simulink model "Attitude"  (R2023b)
settings: Solver=VariableStepAuto  StartTime=0.0  StopTime=10.0  RelTol=1e-3
values from neighbouring files (symbols this model uses):
  gravity = Airplane_data(52)    [Data_edit.m]
libraries: simulink_extras x6, slpidlib x3
settings Model: Creator=saifg  LastModifiedBy=saifg

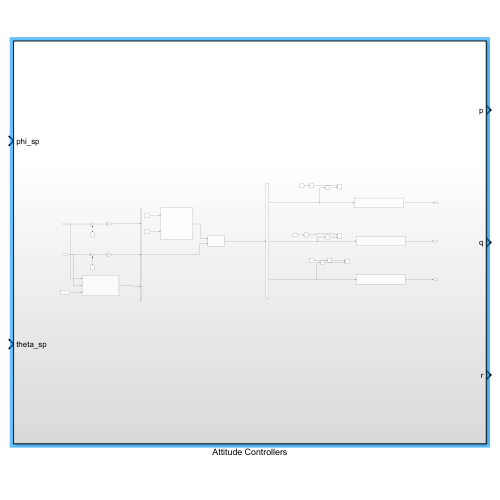
[thumbnail: Simulink's stored preview of the top-level diagram]
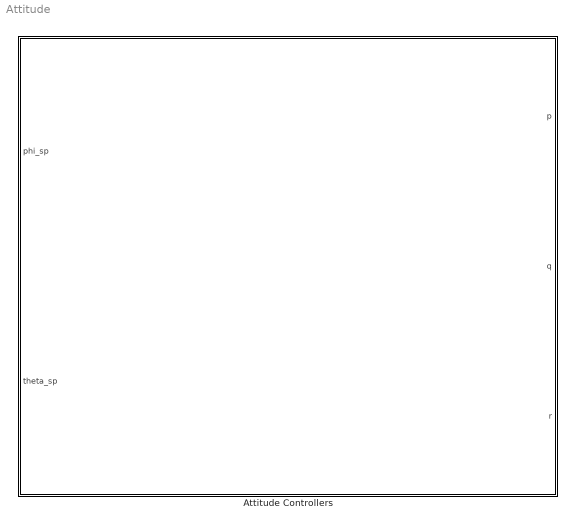
== system Attitude ==
  Attitude Controllers : Subsystem

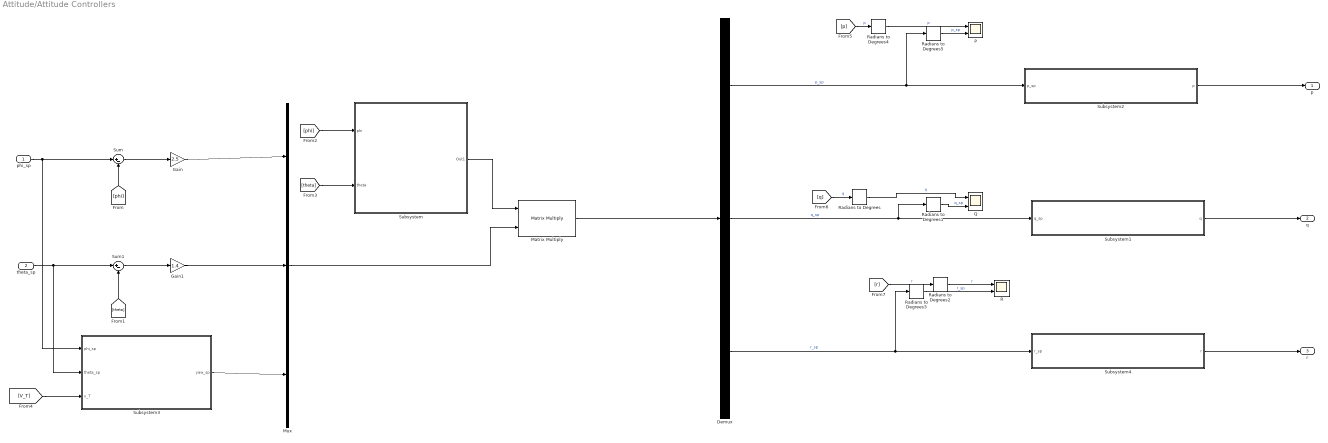
== system Attitude/Attitude Controllers ==
  phi_sp : Inport
  theta_sp : Inport  Port=2
  Demux : Demux  Outputs=3
  Gain : Gain  Gain=2.5
  Gain1 : Gain  Gain=1.4
  Matrix Multiply : Product  Multiplication=Matrix(*)
  Mux : Mux  Inputs=3
  P : Scope  NumInputPorts=2
  Q : Scope  NumInputPorts=2
  R : Scope  NumInputPorts=2
  Radians to Degrees{,1..5} (6 alike) : simulink_extras/Transformations/Radians to Degrees
  Subsystem : Subsystem
  Subsystem1 : Subsystem
  Subsystem2 : Subsystem
  Subsystem3 : Subsystem
  Subsystem4 : Subsystem
  Sum : Sum  Inputs=|+-
  Sum1 : Sum  Inputs=|+-
  p : Outport
  q : Outport  Port=2
  r : Outport  Port=3
  wires:
  [phi] -> Sum/2
  phi_sp/1 -> Subsystem3/1(phi_sp), Sum/1
  Sum/1 -> Gain/1
  theta_sp/1 -> Subsystem3/2(theta_sp), Sum1/1
  [theta] -> Sum1/2
  Sum1/1 -> Gain1/1
  Gain/1 -> Mux/1
  Gain1/1 -> Mux/2
  Subsystem/1(Out1) -> Matrix Multiply/1
  Mux/1 -> Matrix Multiply/2
  Demux/2 -> Radians to Degrees1/1, Subsystem1/1(q_sp)  "q_sp"
  Demux/1 -> Radians to Degrees5/1, Subsystem2/1(p_sp)  "p_sp"
  [phi] -> Subsystem/1(phi)
  [theta] -> Subsystem/2(theta)
  [V_T] -> Subsystem3/3(v_T)
  Subsystem3/1(yaw_sp) -> Mux/3
  Demux/3 -> Radians to Degrees3/1, Subsystem4/1(r_sp)  "r_sp"
  Subsystem2/1(p) -> p/1
  Subsystem1/1(q) -> q/1
  Subsystem4/1(r) -> r/1
  [p] -> Radians to Degrees4/1  "p"
  [q] -> Radians to Degrees/1  "q"
  [r] -> Radians to Degrees2/1  "r"
  Radians to Degrees/1 -> Q/1  "q"
  Radians to Degrees1/1 -> Q/2  "q_sp"
  Radians to Degrees2/1 -> R/1  "r"
  Radians to Degrees3/1 -> R/2  "r_sp"
  Radians to Degrees4/1 -> P/1  "p"
  Radians to Degrees5/1 -> P/2  "p_sp"
  Matrix Multiply/1 -> Demux/1

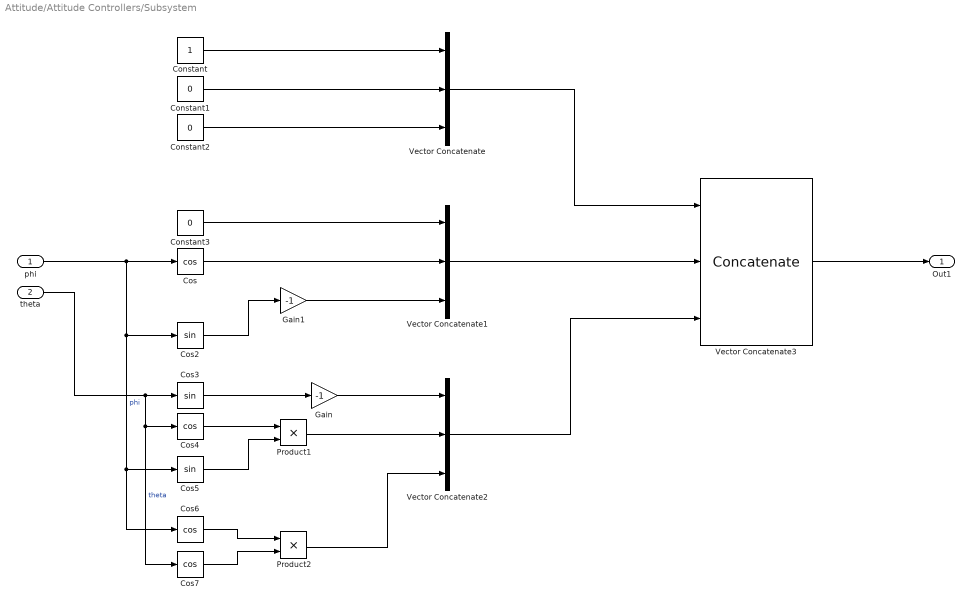
== system Attitude/Attitude Controllers/Subsystem ==
  phi : Inport
  theta : Inport  Port=2
  Constant : Constant
  Constant1 : Constant  Value=0
  Constant2 : Constant  Value=0
  Constant3 : Constant  Value=0
  Cos{,4,6..7} (4 alike) : Trigonometry  Operator=cos
  Cos2 : Trigonometry
  Cos3 : Trigonometry
  Cos5 : Trigonometry
  Gain : Gain  Gain=-1
  Gain1 : Gain  Gain=-1
  Product1 : Product
  Product2 : Product
  Vector Concatenate : Concatenate  NumInputs=3
  Vector Concatenate1 : Concatenate  NumInputs=3
  Vector Concatenate2 : Concatenate  NumInputs=3
  Vector Concatenate3 : Concatenate  NumInputs=3  Mode=Multidimensional array  ConcatenateDimension=2
  Out1 : Outport
  wires:
  Constant2/1 -> Vector Concatenate/3
  Constant1/1 -> Vector Concatenate/2
  Constant/1 -> Vector Concatenate/1
  Constant3/1 -> Vector Concatenate1/1
  Cos/1 -> Vector Concatenate1/2
  Cos2/1 -> Gain1/1
  phi/1 -> Cos6/1, Cos5/1, Cos2/1, Cos/1  "phi"
  theta/1 -> Cos7/1, Cos4/1, Cos3/1  "theta"
  Cos3/1 -> Gain/1
  Gain/1 -> Vector Concatenate2/1
  Cos5/1 -> Product1/2
  Product1/1 -> Vector Concatenate2/2
  Cos4/1 -> Product1/1
  Product2/1 -> Vector Concatenate2/3
  Cos6/1 -> Product2/1
  Cos7/1 -> Product2/2
  Vector Concatenate2/1 -> Vector Concatenate3/3
  Vector Concatenate1/1 -> Vector Concatenate3/2
  Vector Concatenate3/1 -> Out1/1
  Vector Concatenate/1 -> Vector Concatenate3/1
  Gain1/1 -> Vector Concatenate1/3

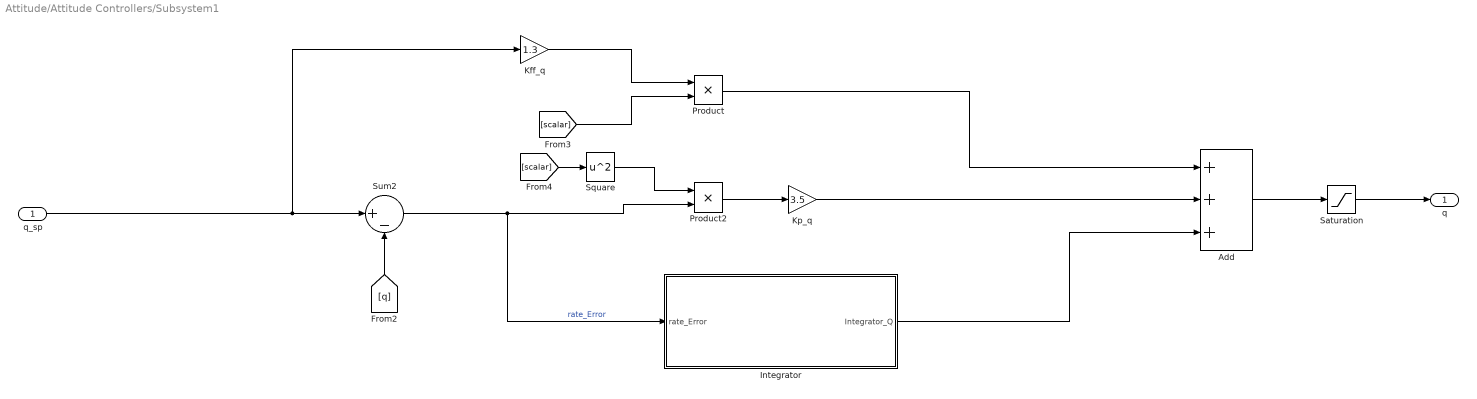
== system Attitude/Attitude Controllers/Subsystem1 ==
  q_sp : Inport
  Add : Sum  Inputs=+++
  Integrator : Subsystem
  Kff_q : Gain  Gain=1.3
  Kp_q : Gain  Gain=3.5
  Product : Product
  Product2 : Product
  Saturation : Saturate  UpperLimit=1  LowerLimit=-1
  Square : Math  Operator=square
  Sum2 : Sum  Inputs=|+-
  q : Outport
  wires:
  Kp_q/1 -> Add/2
  [scalar] -> Product/2
  Square/1 -> Product2/1
  [q] -> Sum2/2
  Kff_q/1 -> Product/1
  q_sp/1 -> Kff_q/1, Sum2/1
  Sum2/1 -> Product2/2, Integrator/1(rate_Error)  "rate_Error"
  [scalar] -> Square/1
  Product2/1 -> Kp_q/1
  Product/1 -> Add/1
  Integrator/1(Integrator_Q) -> Add/3
  Add/1 -> Saturation/1
  Saturation/1 -> q/1

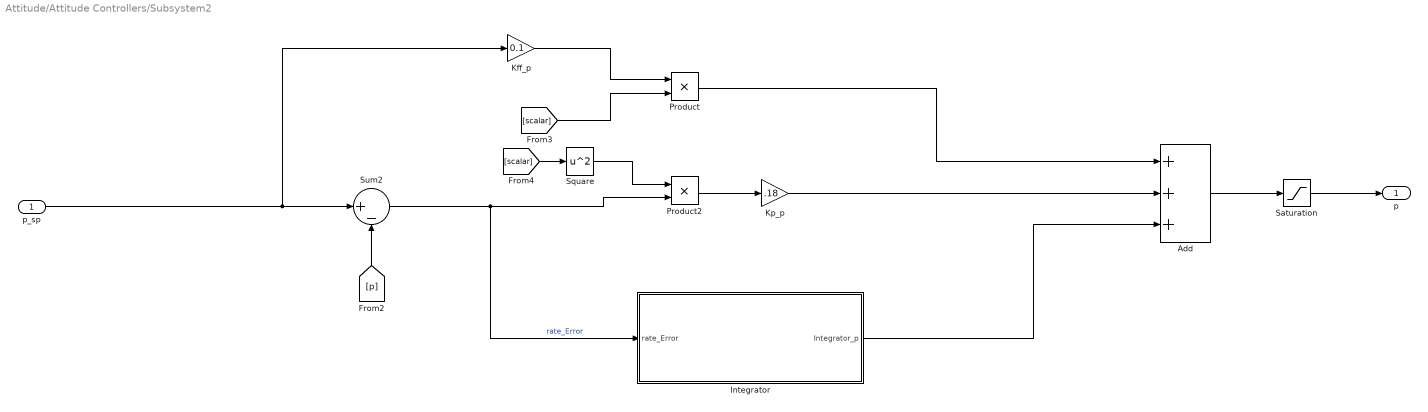
== system Attitude/Attitude Controllers/Subsystem2 ==
  p_sp : Inport
  Add : Sum  Inputs=+++
  Integrator : Subsystem
  Kff_p : Gain  Gain=0.1
  Kp_p : Gain  Gain=.18
  Product : Product
  Product2 : Product
  Saturation : Saturate  UpperLimit=1  LowerLimit=-1
  Square : Math  Operator=square
  Sum2 : Sum  Inputs=|+-
  p : Outport
  wires:
  Add/1 -> Saturation/1
  Integrator/1(Integrator_p) -> Add/3
  Product/1 -> Add/1
  Product2/1 -> Kp_p/1
  [scalar] -> Square/1
  Sum2/1 -> Integrator/1(rate_Error), Product2/2  "rate_Error"
  p_sp/1 -> Sum2/1, Kff_p/1
  Kff_p/1 -> Product/1
  [p] -> Sum2/2
  Square/1 -> Product2/1
  [scalar] -> Product/2
  Kp_p/1 -> Add/2
  Saturation/1 -> p/1

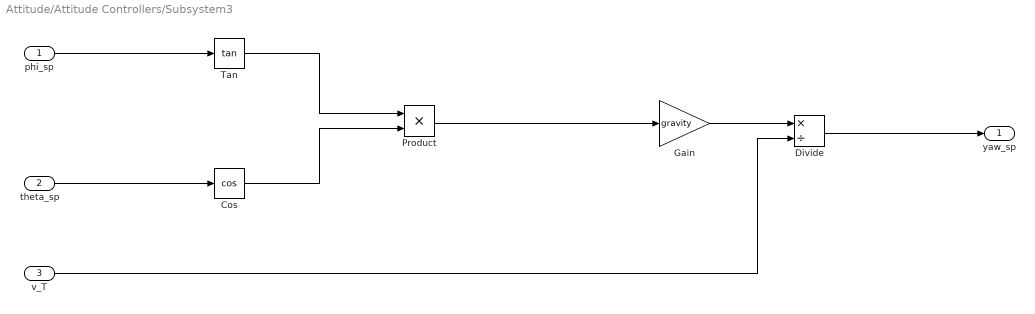
== system Attitude/Attitude Controllers/Subsystem3 ==
  phi_sp : Inport
  theta_sp : Inport  Port=2
  v_T : Inport  Port=3
  Cos : Trigonometry  Operator=cos
  Divide : Product  Inputs=*/
  Gain : Gain  Gain=gravity
  Product : Product
  Tan : Trigonometry  Operator=tan
  yaw_sp : Outport
  wires:
  phi_sp/1 -> Tan/1
  theta_sp/1 -> Cos/1
  Cos/1 -> Product/2
  Tan/1 -> Product/1
  Product/1 -> Gain/1
  Gain/1 -> Divide/1
  v_T/1 -> Divide/2
  Divide/1 -> yaw_sp/1

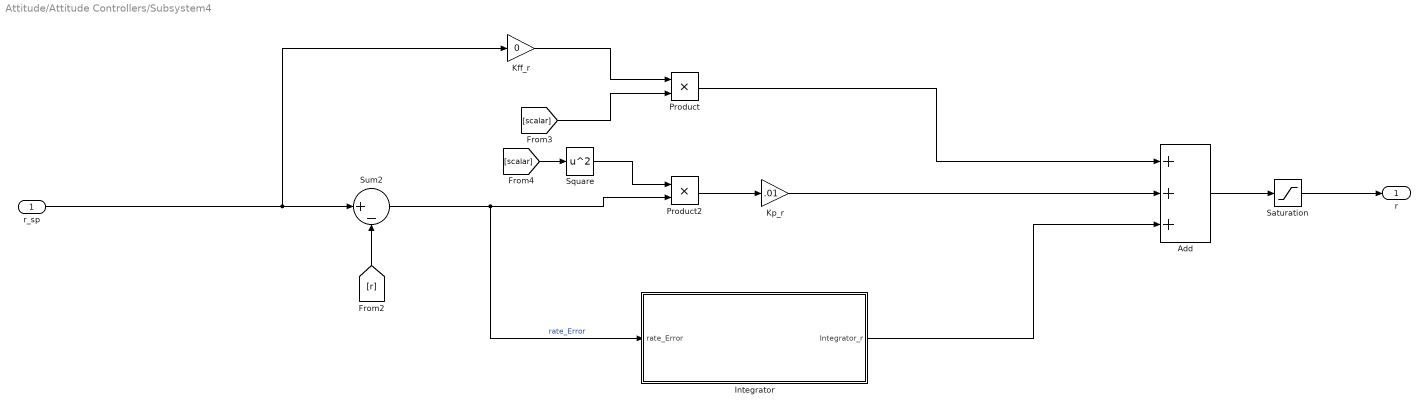
== system Attitude/Attitude Controllers/Subsystem4 ==
  r_sp : Inport
  Add : Sum  Inputs=+++
  Integrator : Subsystem
  Kff_r : Gain  Gain=0
  Kp_r : Gain  Gain=.01
  Product : Product
  Product2 : Product
  Saturation : Saturate  UpperLimit=1  LowerLimit=-1
  Square : Math  Operator=square
  Sum2 : Sum  Inputs=|+-
  r : Outport
  wires:
  Add/1 -> Saturation/1
  Integrator/1(Integrator_r) -> Add/3
  Product/1 -> Add/1
  Product2/1 -> Kp_r/1
  [scalar] -> Square/1
  Sum2/1 -> Integrator/1(rate_Error), Product2/2  "rate_Error"
  r_sp/1 -> Sum2/1, Kff_r/1
  Kff_r/1 -> Product/1
  [r] -> Sum2/2
  Square/1 -> Product2/1
  Kp_r/1 -> Add/2
  Saturation/1 -> r/1
  [scalar] -> Product/2

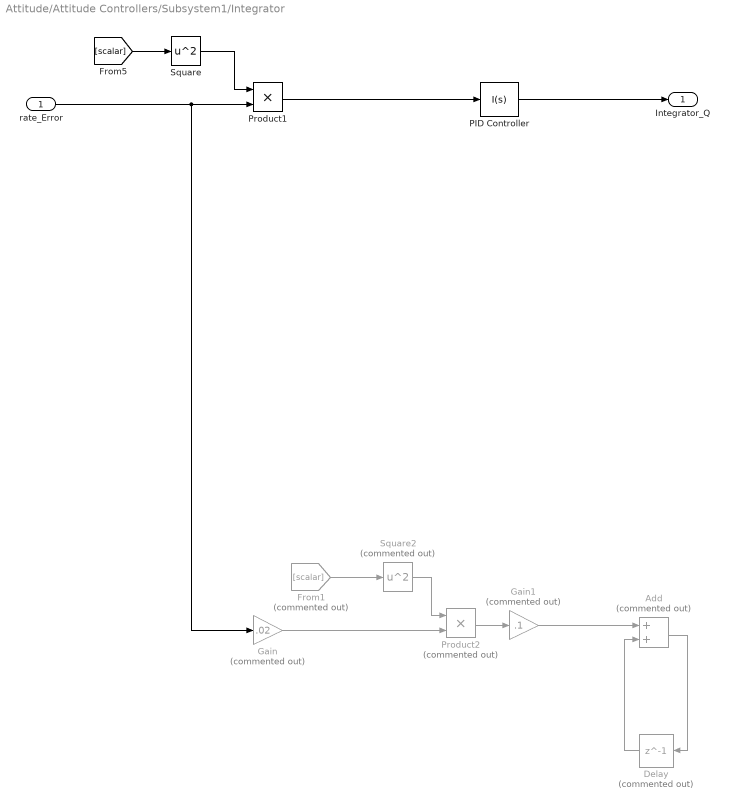
== system Attitude/Attitude Controllers/Subsystem1/Integrator ==
  rate_Error : Inport
  Add : Sum  Commented=on
  Delay : Delay  Commented=on  DelayLength=1
  From1 : From  Commented=on  GotoTag=scalar  TagVisibility=global
  Gain : Gain  Commented=on  Gain=.02
  Gain1 : Gain  Commented=on  Gain=.1
  PID Controller : slpidlib/PID Controller  Controller=I  Form=Parallel  TimeDomain=Continuous-time  UseExternalTs=off  SampleTime=-1  IntegratorMethod=Forward Euler  FilterMethod=Forward Euler  ControllerParametersSource=internal  P=0  I=1.2  UseKiTs=off  D=0  N=100  UseFilter=on  TunerSelectOption=Transfer Function Based (PID Tuner App)  InitialConditionSource=internal  InitialConditionForIntegrator=0  InitialConditionForFilter=0  DifferentiatorICPrevScaledInput=0  ExternalReset=none  TrackingMode=off  Kt=1  LimitOutput=on  SatLimitsSource=internal  UpperSaturationLimit=0.4000000059604645  LowerSaturationLimit=-0.4000000059604645  LinearizeAsGain=on  AntiWindupMode=back-calculation  Kb=0.4  LimitIntegrator=off  UpperIntegratorSaturationLimit=inf  LowerIntegratorSaturationLimit=-inf  POutMin=[]  POutMax=[]  IOutMin=[]  IOutMax=[]  DOutMin=[]  DOutMax=[]  NOutMin=[]  NOutMax=[]  SumOutMin=[]  SumOutMax=[]  SaturationOutMin=[]  SaturationOutMax=[]  PParamMin=[]  PParamMax=[]  IParamMin=[]  IParamMax=[]  DParamMin=[]  DParamMax=[]  NParamMin=[]  NParamMax=[]  KbParamMin=[]  KbParamMax=[]  KtParamMin=[]  KtParamMax=[]  KbOutMin=[]  KbOutMax=[]  KtOutMin=[]  KtOutMax=[]  IntegratorOutMin=[]  IntegratorOutMax=[]  FilterOutMin=[]  FilterOutMax=[]  SumI1OutMin=[]  SumI1OutMax=[]  SumI2OutMin=[]  SumI2OutMax=[]  SumI3OutMin=[]  SumI3OutMax=[]  SumI4OutMin=[]  SumI4OutMax=[]  SumDOutMin=[]  SumDOutMax=[]  DifferentiatorOutMin=[]  DifferentiatorOutMax=[]  FilterDiffOutCoefMin=[]  FilterDiffOutCoefMax=[]  ReciprocalOutMin=[]  ReciprocalOutMax=[]  SumDenOutMin=[]  SumDenOutMax=[]  SumNumOutMin=[]  SumNumOutMax=[]  DivideOutMin=[]  DivideOutMax=[]  UdiffTsProdOutMin=[]  UdiffTsProdOutMax=[]  NTsProdOutMin=[]  NTsProdOutMax=[]  UintegralTsProdOutMin=[]  UintegralTsProdOutMax=[]  UngainTsProdOutMin=[]  UngainTsProdOutMax=[]  ClampingZeroOutDataTypeStr=Inherit: Inherit via back propagation  ClampingZeroOutMin=[]  ClampingZeroOutMax=[]  FilterDenConstantOutDataTypeStr=Inherit: Inherit via back propagation  FilterDenConstantOutMin=[]  FilterDenConstantOutMax=[]  PCopyOutDataTypeStr=Inherit: Inherit via back propagation  PCopyOutMin=[]  PCopyOutMax=[]  NCopyOutDataTypeStr=Inherit: Inherit via back propagation  NCopyOutMin=[]  NCopyOutMax=[]  IntegratorContinuousStateAttributes=''  IntegratorStateMustResolveToSignalObject=off  IntegratorRTWStateStorageClass=Auto  FilterContinuousStateAttributes=''  FilterStateMustResolveToSignalObject=off  FilterRTWStateStorageClass=Auto  ParallelPVariant=Disabled  IdealPVariant=Disabled  IVariant=InternalParameters  DVariant=Disabled  IntegratorVariant=Continuous  SatVariant=Enabled  AWVariant=BackCalculation  PCopyVariant=Disabled  TRVariant=Disabled  FdbkBlocksVariant=Forward  IdealPFdbkVariant=Disabled  SatFdbkVariant=Disabled  DerivativeFilterVariant=Disabled  NVariant=Disabled  NCopyVariant=Disabled_SignalSpec  FilterICVariant=Disabled  IntegratorICVariant=InternalICs  ExternalResetVariant=Disabled  TRSumVariant=Passthrough  SumFdbkVariant=Disabled  SumVariant=Passthrough_I  TsampFilterVariant=InternalTs  TsampNgainVariant=Passthrough  TsampIntegralVariant=Disabled_SignalSpec  ExternalSaturationOutDataTypeStr=Inherit: Same as second input
  Product1 : Product
  Product2 : Product  Commented=on
  Square : Math  Operator=square
  Square2 : Math  Commented=on  Operator=square
  Integrator_Q : Outport
  wires:
  Product1/1 -> PID Controller/1
  [scalar] -> Square/1
  rate_Error/1 -> Gain/1, Product1/2
  Gain/1 -> Product2/2
  Square2/1 -> Product2/1
  From1/1 -> Square2/1
  Product2/1 -> Gain1/1
  Add/1 -> Delay/1
  Delay/1 -> Add/2
  Gain1/1 -> Add/1
  PID Controller/1 -> Integrator_Q/1
  Square/1 -> Product1/1

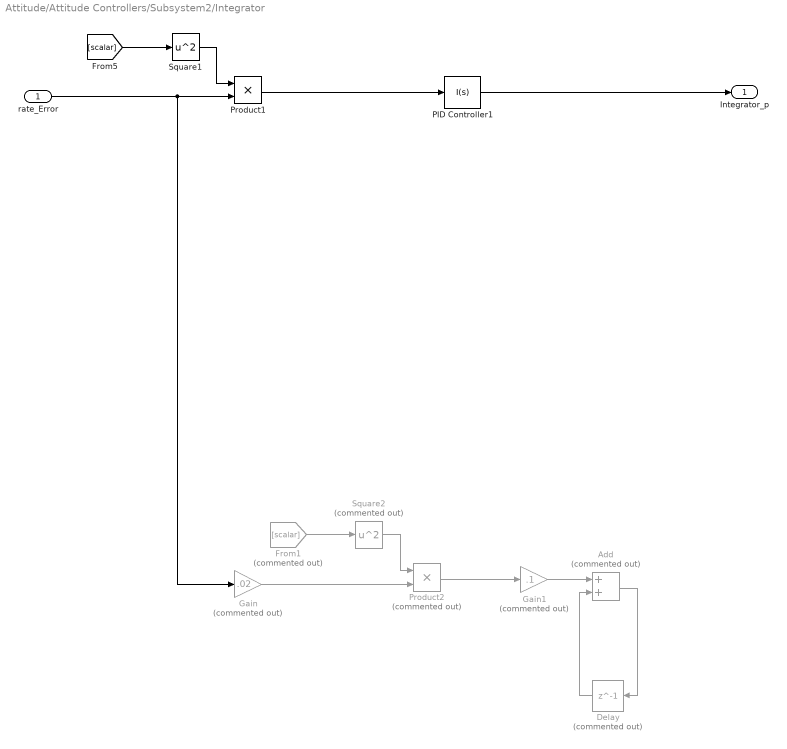
== system Attitude/Attitude Controllers/Subsystem2/Integrator ==
  rate_Error : Inport
  Add : Sum  Commented=on
  Delay : Delay  Commented=on  DelayLength=1
  From1 : From  Commented=on  GotoTag=scalar  TagVisibility=global
  Gain : Gain  Commented=on  Gain=.02
  Gain1 : Gain  Commented=on  Gain=.1
  PID Controller1 : slpidlib/PID Controller  Controller=I  Form=Parallel  TimeDomain=Continuous-time  UseExternalTs=off  SampleTime=-1  IntegratorMethod=Forward Euler  FilterMethod=Forward Euler  ControllerParametersSource=internal  P=0  I=0.1  UseKiTs=off  D=0  N=100  UseFilter=on  TunerSelectOption=Transfer Function Based (PID Tuner App)  InitialConditionSource=internal  InitialConditionForIntegrator=0  InitialConditionForFilter=0  DifferentiatorICPrevScaledInput=0  ExternalReset=none  TrackingMode=off  Kt=1  LimitOutput=on  SatLimitsSource=internal  UpperSaturationLimit=0.20000000298023224  LowerSaturationLimit=-0.20000000298023224  LinearizeAsGain=on  AntiWindupMode=back-calculation  Kb=0.2  LimitIntegrator=off  UpperIntegratorSaturationLimit=inf  LowerIntegratorSaturationLimit=-inf  POutMin=[]  POutMax=[]  IOutMin=[]  IOutMax=[]  DOutMin=[]  DOutMax=[]  NOutMin=[]  NOutMax=[]  SumOutMin=[]  SumOutMax=[]  SaturationOutMin=[]  SaturationOutMax=[]  PParamMin=[]  PParamMax=[]  IParamMin=[]  IParamMax=[]  DParamMin=[]  DParamMax=[]  NParamMin=[]  NParamMax=[]  KbParamMin=[]  KbParamMax=[]  KtParamMin=[]  KtParamMax=[]  KbOutMin=[]  KbOutMax=[]  KtOutMin=[]  KtOutMax=[]  IntegratorOutMin=[]  IntegratorOutMax=[]  FilterOutMin=[]  FilterOutMax=[]  SumI1OutMin=[]  SumI1OutMax=[]  SumI2OutMin=[]  SumI2OutMax=[]  SumI3OutMin=[]  SumI3OutMax=[]  SumI4OutMin=[]  SumI4OutMax=[]  SumDOutMin=[]  SumDOutMax=[]  DifferentiatorOutMin=[]  DifferentiatorOutMax=[]  FilterDiffOutCoefMin=[]  FilterDiffOutCoefMax=[]  ReciprocalOutMin=[]  ReciprocalOutMax=[]  SumDenOutMin=[]  SumDenOutMax=[]  SumNumOutMin=[]  SumNumOutMax=[]  DivideOutMin=[]  DivideOutMax=[]  UdiffTsProdOutMin=[]  UdiffTsProdOutMax=[]  NTsProdOutMin=[]  NTsProdOutMax=[]  UintegralTsProdOutMin=[]  UintegralTsProdOutMax=[]  UngainTsProdOutMin=[]  UngainTsProdOutMax=[]  ClampingZeroOutDataTypeStr=Inherit: Inherit via back propagation  ClampingZeroOutMin=[]  ClampingZeroOutMax=[]  FilterDenConstantOutDataTypeStr=Inherit: Inherit via back propagation  FilterDenConstantOutMin=[]  FilterDenConstantOutMax=[]  PCopyOutDataTypeStr=Inherit: Inherit via back propagation  PCopyOutMin=[]  PCopyOutMax=[]  NCopyOutDataTypeStr=Inherit: Inherit via back propagation  NCopyOutMin=[]  NCopyOutMax=[]  IntegratorContinuousStateAttributes=''  IntegratorStateMustResolveToSignalObject=off  IntegratorRTWStateStorageClass=Auto  FilterContinuousStateAttributes=''  FilterStateMustResolveToSignalObject=off  FilterRTWStateStorageClass=Auto  ParallelPVariant=Disabled  IdealPVariant=Disabled  IVariant=InternalParameters  DVariant=Disabled  IntegratorVariant=Continuous  SatVariant=Enabled  AWVariant=BackCalculation  PCopyVariant=Disabled  TRVariant=Disabled  FdbkBlocksVariant=Forward  IdealPFdbkVariant=Disabled  SatFdbkVariant=Disabled  DerivativeFilterVariant=Disabled  NVariant=Disabled  NCopyVariant=Disabled_SignalSpec  FilterICVariant=Disabled  IntegratorICVariant=InternalICs  ExternalResetVariant=Disabled  TRSumVariant=Passthrough  SumFdbkVariant=Disabled  SumVariant=Passthrough_I  TsampFilterVariant=InternalTs  TsampNgainVariant=Passthrough  TsampIntegralVariant=Disabled_SignalSpec  ExternalSaturationOutDataTypeStr=Inherit: Same as second input
  Product1 : Product
  Product2 : Product  Commented=on
  Square1 : Math  Operator=square
  Square2 : Math  Commented=on  Operator=square
  Integrator_p : Outport
  wires:
  Delay/1 -> Add/2
  Add/1 -> Delay/1
  Product2/1 -> Gain1/1
  From1/1 -> Square2/1
  Square2/1 -> Product2/1
  Gain/1 -> Product2/2
  rate_Error/1 -> Product1/2, Gain/1
  Square1/1 -> Product1/1
  [scalar] -> Square1/1
  Gain1/1 -> Add/1
  Product1/1 -> PID Controller1/1
  PID Controller1/1 -> Integrator_p/1

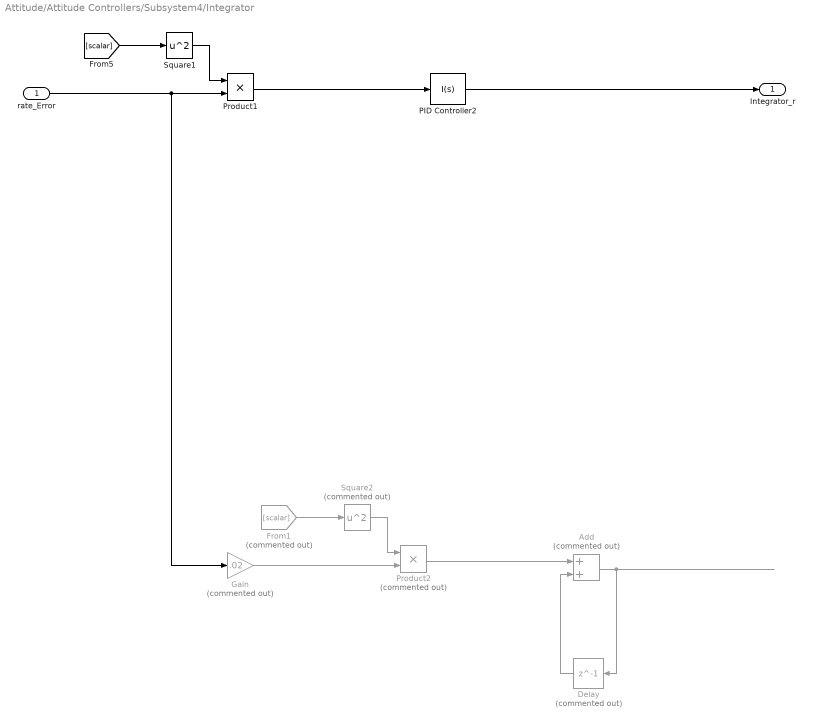
== system Attitude/Attitude Controllers/Subsystem4/Integrator ==
  rate_Error : Inport
  Add : Sum  Commented=on
  Delay : Delay  Commented=on  DelayLength=1
  From1 : From  Commented=on  GotoTag=scalar
  Gain : Gain  Commented=on  Gain=.02
  PID Controller2 : slpidlib/PID Controller  Controller=I  Form=Parallel  TimeDomain=Continuous-time  UseExternalTs=off  SampleTime=-1  IntegratorMethod=Forward Euler  FilterMethod=Forward Euler  ControllerParametersSource=internal  P=0  I=0.1  UseKiTs=off  D=0  N=100  UseFilter=on  TunerSelectOption=Transfer Function Based (PID Tuner App)  InitialConditionSource=internal  InitialConditionForIntegrator=0  InitialConditionForFilter=0  DifferentiatorICPrevScaledInput=0  ExternalReset=none  TrackingMode=off  Kt=1  LimitOutput=on  SatLimitsSource=internal  UpperSaturationLimit=0.20000000298023224  LowerSaturationLimit=-0.20000000298023224  LinearizeAsGain=on  AntiWindupMode=back-calculation  Kb=0.8  LimitIntegrator=off  UpperIntegratorSaturationLimit=inf  LowerIntegratorSaturationLimit=-inf  POutMin=[]  POutMax=[]  IOutMin=[]  IOutMax=[]  DOutMin=[]  DOutMax=[]  NOutMin=[]  NOutMax=[]  SumOutMin=[]  SumOutMax=[]  SaturationOutMin=[]  SaturationOutMax=[]  PParamMin=[]  PParamMax=[]  IParamMin=[]  IParamMax=[]  DParamMin=[]  DParamMax=[]  NParamMin=[]  NParamMax=[]  KbParamMin=[]  KbParamMax=[]  KtParamMin=[]  KtParamMax=[]  KbOutMin=[]  KbOutMax=[]  KtOutMin=[]  KtOutMax=[]  IntegratorOutMin=[]  IntegratorOutMax=[]  FilterOutMin=[]  FilterOutMax=[]  SumI1OutMin=[]  SumI1OutMax=[]  SumI2OutMin=[]  SumI2OutMax=[]  SumI3OutMin=[]  SumI3OutMax=[]  SumI4OutMin=[]  SumI4OutMax=[]  SumDOutMin=[]  SumDOutMax=[]  DifferentiatorOutMin=[]  DifferentiatorOutMax=[]  FilterDiffOutCoefMin=[]  FilterDiffOutCoefMax=[]  ReciprocalOutMin=[]  ReciprocalOutMax=[]  SumDenOutMin=[]  SumDenOutMax=[]  SumNumOutMin=[]  SumNumOutMax=[]  DivideOutMin=[]  DivideOutMax=[]  UdiffTsProdOutMin=[]  UdiffTsProdOutMax=[]  NTsProdOutMin=[]  NTsProdOutMax=[]  UintegralTsProdOutMin=[]  UintegralTsProdOutMax=[]  UngainTsProdOutMin=[]  UngainTsProdOutMax=[]  ClampingZeroOutDataTypeStr=Inherit: Inherit via back propagation  ClampingZeroOutMin=[]  ClampingZeroOutMax=[]  FilterDenConstantOutDataTypeStr=Inherit: Inherit via back propagation  FilterDenConstantOutMin=[]  FilterDenConstantOutMax=[]  PCopyOutDataTypeStr=Inherit: Inherit via back propagation  PCopyOutMin=[]  PCopyOutMax=[]  NCopyOutDataTypeStr=Inherit: Inherit via back propagation  NCopyOutMin=[]  NCopyOutMax=[]  IntegratorContinuousStateAttributes=''  IntegratorStateMustResolveToSignalObject=off  IntegratorRTWStateStorageClass=Auto  FilterContinuousStateAttributes=''  FilterStateMustResolveToSignalObject=off  FilterRTWStateStorageClass=Auto  ParallelPVariant=Disabled  IdealPVariant=Disabled  IVariant=InternalParameters  DVariant=Disabled  IntegratorVariant=Continuous  SatVariant=Enabled  AWVariant=BackCalculation  PCopyVariant=Disabled  TRVariant=Disabled  FdbkBlocksVariant=Forward  IdealPFdbkVariant=Disabled  SatFdbkVariant=Disabled  DerivativeFilterVariant=Disabled  NVariant=Disabled  NCopyVariant=Disabled_SignalSpec  FilterICVariant=Disabled  IntegratorICVariant=InternalICs  ExternalResetVariant=Disabled  TRSumVariant=Passthrough  SumFdbkVariant=Disabled  SumVariant=Passthrough_I  TsampFilterVariant=InternalTs  TsampNgainVariant=Passthrough  TsampIntegralVariant=Disabled_SignalSpec  ExternalSaturationOutDataTypeStr=Inherit: Same as second input
  Product1 : Product
  Product2 : Product  Commented=on
  Square1 : Math  Operator=square
  Square2 : Math  Commented=on  Operator=square
  Integrator_r : Outport
  wires:
  Delay/1 -> Add/2
  Add/1 -> Delay/1
  Product2/1 -> Add/1
  From1/1 -> Square2/1
  Square2/1 -> Product2/1
  Gain/1 -> Product2/2
  rate_Error/1 -> Product1/2, Gain/1
  Square1/1 -> Product1/1
  Product1/1 -> PID Controller2/1
  [scalar] -> Square1/1
  PID Controller2/1 -> Integrator_r/1
